simulink subsystem "connector"  (R2023a)
settings: Solver=VariableStepAuto  StartTime=0.0  StopTime=10.0  RelTol=1e-3
model mask{k1=0, k2=0, k3=0}
  mask prompts: k1 "Значение постоянного напряжения"; k2 "Значение амплитуды синусоидального регулирования напряжения"; k3 "Значение амплитуды ШИМ регулирования напряжения"
settings Model: Creator=diontep  LastModifiedBy=diontep

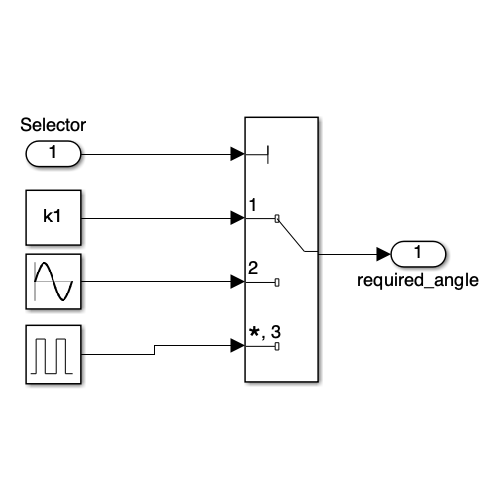
[thumbnail: Simulink's stored preview of the top-level diagram]
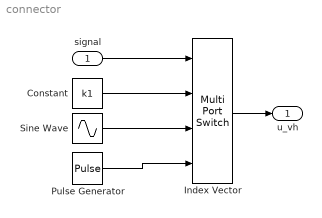
== system connector ==
  "signal " : Inport
  Constant : Constant  Value=k1
  Index Vector : MultiPortSwitch  SaturateOnIntegerOverflow=off  InputSameDT=off
  Pulse Generator : DiscretePulseGenerator  PulseType=Time based  Amplitude=k3  Period=0.1  PulseWidth=5
  Sine Wave : Sin  Amplitude=k2  SampleTime=0
  u_vh : Outport
  wires:
  Index Vector/1 -> u_vh/1
  Sine Wave/1 -> Index Vector/3
  "signal "/1 -> Index Vector/1
  Constant/1 -> Index Vector/2
  Pulse Generator/1 -> Index Vector/4
